simulink model "Prob1DynVibrAbs"  (R2019b)
settings: Solver=VariableStepAuto  StartTime=0  StopTime=10.0  MaxStep=0.001  RelTol=1e-3
model workspace (MAT data in the model file):
  K12 = Simulink.Parameter
  K12.Value = 50
  K12.DataType = 'auto'
  K12.Dimensions = [1 1]
  M2 = Simulink.Parameter
  M2.Value = 75
  M2.DataType = 'auto'
  M2.Dimensions = [1 1]
settings Model: Creator=ip  LastModifiedBy=ip

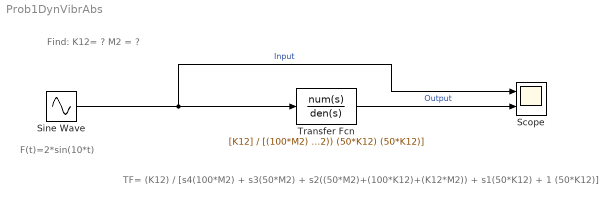
== system Prob1DynVibrAbs ==
  note: Find:
      | K12= ?
      | M2 = ?
  note: TF= (K12) / [s4(100*M2) + s3(50*M2) + s2((50*M2)+(100*K12)+(K12*M2)) + s1(50*K12) + 1 (50*K12)]
  note: F(t)=2*sin(10*t)
  Scope : Scope  NumInputPorts=2
  Sine Wave : Sin  Amplitude=2  Frequency=10  SampleTime=0
  Transfer Fcn : TransferFcn  Numerator=[K12]  Denominator=[(100*M2) (50*M2) ((50*M2)+(100*K12)+(K12*M2)) (50*K12) (50*K12)]
  wires:
  Sine Wave/1 -> Scope/1, Transfer Fcn/1  "Input"
  Transfer Fcn/1 -> Scope/2  "Output"
